simulink model "HevMmPowertrainController"  (R2021b)
settings: Solver=VariableStepAuto  StartTime=0.0  StopTime=inf  FixedStep=.01  RelTol=1e-3  EnableMultiTasking=on
model workspace (MAT data in the model file):
  Active_Scenario_Index = 1
  BattChrgMax = -105500
  BattDischrgMax = 211000
  BattTempInit = 25
  Battery.SOC_LUT = [0.01 0.02 0.03 0.04 0.05 0.06 0.07 0.08 0.09 0.1 0.11 0.12 0.13 0.14 0.15 0.16 0.17 0.18 0.19 0.2 0.21 0.22 0.23 0.24 0.25 0.26 0.27 0.28 0.29 0.3 0.31 0.32 0.33 0.34 0.35 0.36 0.37 0.38 0.39 0.4 0.41 0.42 0.43 0.44 0.45 0.46 0.47 0.48 0.49 0.5 0.51 0.52 0.53 0.54 0.55 0.56 0.57 0.58 0.59 0.6 0.61 0.62 0.63 0.64 0.65 0.66 0.67 0.68 0.69 0.7 0.71 0.72 0.73 0.74 0.75 0.76 0.77 0.78 0.79 0.8 0.81 0.82 0.83 0.84 0.85 0.86 0.87 0.88 0.89 0.9 0.91 0.92 0.93 0.94 0.95 0.96 0.97 0.98 0.99 1]
  Battery.Temperature_LUT = [-10 0 25 40]
  Battery.Capacity_LUT = [4.04528301887 4.19622641509 4.8 4.73962264151]
  Battery.Em_LUT = [2.67308083891 2.74411674384 2.80408613071 2.86247711994 2.90851059763 2.94904306488 2.9829846776 3.01467102589 3.04031502638 3.06256828113 3.08180972392 3.09994219643 ... (400 elements, 100x4)]
  Battery.R0_LUT = [0.0569026752707 0.0575506938969 0.0576730924021 0.0575627404981 0.0573787336615 0.0571931123197 0.0568199985482 0.056411926464 0.0561974340667 0.0560805640861 0.0557640899305 0.055275807865 ... (400 elements, 100x4)]
  Battery.R1_LUT = [0.0035 0.0035 0.0035 0.0035 0.0035 0.0035 0.0035 0.0035 0.0035 0.0035 0.0035 0.0035 ... (400 elements, 100x4)]
  Battery.C1_LUT = [5000 5000 5000 5000 5000 5000 5000 5000 5000 5000 5000 5000 ... (400 elements, 100x4)]
  Battery.Mass = 0.047
  Battery.ThermalMass = 44
  Battery.R_bleed = 20
  Battery.h_conv = 5
  Battery.cell_area = 0.0037
  Battery.TempInit = 25
  Battery.SOCInit = 0.75
  Battery.Model = 'panasonic ncr18650bd'
  Battery.DischargeCycle_LUT = [1 5 9 13 17 21 25 29 33 37 41 45 49 53 57 61 65 69 73 77 81 85 89 93 97 101 105 109 113 117 121 125 129 133 137 141 145 149 153 157 161 165 169 173 177 181 185 189 193 197 201 205 209 213 217 221 225 229 233 237 241 245 249 253 257 261 265 269 273 277 281 285 289 293 297 301 305 309 313 317]
  Battery.deltaEm_LUT = [0 -0.363115641304 -0.600096647258 -0.689070000839 -0.76773380251 -0.846397604181 -0.926368385458 -0.992711297521 -1.05704974111 -1.12227693902 -1.19018070587 -1.25808447272 -1.31699459748 -1.35876443799 -1.40168267642 -1.44460091485 -1.48751915327 -1.5304373917 -1.57335563013 -1.62198241593 -1.67232184498 -1.71858340023 -1.76179802551 -1.8050126508 -1.84822727608 -1.8917937136 -1.93575272784 -1.97971174208 -2.02367075632 -2.06762977056 -2.11171979109 -2.15588700406 -2.19980020032 -2.24365853098 -2.28751686164 -2.33137519231 -2.37523352297 -2.41909185363 -2.45982559031 -2.49599372373 -2.53216185715 -2.56832999058 -2.604498124 -2.64066625743 -2.67683439085 -2.71300252428 -2.7491706577 -2.78367585394 -2.81632179346 -2.8483348579 -2.88034792233 -2.91236098677 -2.94437405121 -2.97638711564 -3.00840018008 -3.04041324451 -3.07260346059 -3.10359008254 -3.13082308991 -3.15805609728 -3.18528910464 -3.21252211201 -3.23975511938 -3.26698812675 -3.29422113412 -3.32122400938 -3.3463475604 -3.37152613073 -3.39670470105 -3.42188327138 -3.4470618417 -3.47224041203 -3.49938358795 -3.52900276724 -3.55862194653 -3.58824112582 -3.6178603051 -3.64748858268 -3.67711690909 -3.70674523549]
  Battery.deltaCapacity_LUT = [0 -0.860019120059 -1.71332421702 -2.0819400264 -2.45055583577 -2.81917164515 -3.18778745452 -3.48884924257 -3.7808148236 -4.07278040463 -4.36474598566 -4.6567115667 -4.91000721732 -5.08494410056 -5.2598809838 -5.43481786703 -5.60975475027 -5.78469163351 -5.95962851674 -6.13456539998 -6.30950228322 -6.47026795816 -6.62044510558 -6.77062225299 -6.92079940041 -7.07097654783 -7.22115369524 -7.37133084266 -7.52150799007 -7.67168513749 -7.82230984162 -7.97319825819 -8.12408667477 -8.27497509134 -8.42586350792 -8.57675192449 -8.72764034107 -8.87852875764 -9.01789522921 -9.13717923376 -9.25646323831 -9.37574724285 -9.4950312474 -9.61431525195 -9.73359925649 -9.85288326104 -9.97216726558 -10.0914512701 -10.2059878191 -10.3183039593 -10.4306200996 -10.5429362398 -10.65525238 -10.7675685203 -10.8798846605 -10.9922008008 -11.104516941 -11.2125891929 -11.3075699376 -11.4025506823 -11.4975314271 -11.5925121718 -11.6874929166 -11.7824736613 -11.877454406 -11.9716325175 -12.0588579537 -12.1460833899 -12.2333088261 -12.3205342623 -12.4077596986 -12.4949851348 -12.5890165008 -12.6916254178 -12.7942343349 -12.8968432519 -12.999452169 -13.102061086 -13.2046700031 -13.3072789201]
  Battery.cond_thickness = 0.001
  Battery.thermal_conductivity = 205
  BrkPrsMax = 5000000
  CellType = 1
  ChrgLmt_bpt = [1 1 1 1 1 1 1 1 0.7 0.35 0]
  ChrgSOCHi = 80
  ChrgSOCLo = 70
  DischrgLmt_bpt = [0 0.35 0.7 1 1 1 1 1 1 1 1]
  EngCltchOffTractiveForce = 3000
  EngCltchOffVehSpd = 70
  EngCltchOnTractiveForce = 2000
  EngCltchOnVehSpd = 80
  EngCltchOnWait = 5
  EngDriveRatio = 2
  FricBrakeCmd = [0 0 12 24 36 48 60]
  FricBrakeCmdBpt = [0 0.1 0.2 0.4 0.6 0.8 1]
  MaxChrgPwr = 50000
  MaxRegenPwr = 10000
  MotGbRatio = 2.45
  MotMapEff = 0
  MotSpd = [0 1600 3200 4477.56 4800 6400 8000 9600 11200 12800 14400 16000]
  MotTrq = [450 450 450 450 419.771162405 314.828371804 251.862697443 209.885581202 179.901926745 157.414185902 139.923720802 125.931348721]
  Ndiff = 3.421
  Np_Module = 31
  Ns_Module = 24
  NumModules = 4
  OverCellVoltageLimit = 4.19999980927
  RegenBrkCutOff = [0 1]
  RegenBrkSpd_bpt = [5 9]
  Rm = 0.17778
  SOC_bpt = [0 10 20 30 40 50 60 70 80 90 100]
  T_eff_bp = [0 32.1428571429 64.2857142857 96.4285714286 128.571428571 160.714285714 192.857142857 225 257.142857143 289.285714286 321.428571429 353.571428571 385.714285714 417.857142857 450]
  TestCase = 1
  Ts = 0.01
  UnderCellVoltageLimit = 2.5
  disk_abore = 0.05
  efficiency_table = [86.7  86.7  86.7  86.7  86.7  86.7  86.7  86.7  86.7  86.7  86.7  86.7  86.7  86.7  86.7; 86.7  86.7  86.7  86.7  86.7  86.7  86.7  86.7  86.7  86.7  86.7  86.7  86.7  86.7  86.7; 86.7  86.7  91.8  91.8  91.8  91.8  91.8  91.8  91.8  91.8  89.76  89.76  89.76  89.76  89.76; 86.7  86.7  93.84  93.84  93.84  93.84  93.84  93.84  93.84  93.84  93.84  91.8  91.8  91.8  91.8; 86.7  86.7  93.84  93.84  94.86  94.86  94.86  94.86  93.84  93.84  93.84  91.8  91.8  91.8  91.8; 86.7  86.7  94.86  95.88  95.88  95.88  95.88  95.88  95.88  95.88  95.88  95.88  95.88  95.88  95.88; 86.7  86.7  94.86  95.88  95.88  96.9  96.9  96.9  96.9  96.9  96.9  96.9  96.9  96.9  96.9; 86.7  86.7  94.86  95.88  95.88  96.9  96.9  96.9  96.9  96.9  96.9  96.9  96.9  96.9  96.9; 86.7  86.7  94.86  95.88  96.9  96.9  96.9  96.9  96.9  96.9  96.9  96.9  96.9  96.9  96.9; 86.7  86.7  94.86  95.88  96.9  96.9  96.9  96.9  96.9  96.9  96.9  96.9  96.9  96.9  96.9; 86.7  86.7  94.86  95.88  95.88  95.88  95.88  95.88  95.88  95.88  95.88  95.88  95.88  95.88  95.88; 86.7  86.7  91.8  93.84  94.86  94.86  94.86  94.86  94.86  94.86  94.86  94.86  94.86  94.86  94.86]
  eng.pwr = [15052.6315789 19736.8421053 24421.0526316 29105.2631579 33789.4736842 38473.6842105 43157.8947368 47842.1052632 52526.3157895 57210.5263158 61894.7368421 66578.9473684 71263.1578947 75947.3684211 80631.5789474 85315.7894737 90000]
  eng.spd = [1448.84862461 1712.99052669 1980.33600187 2249.1155588 2517.55970613 2783.89895252 3046.3638066 3303.18477703 3552.59237246 3792.81710154 4022.08947291 4238.63999523 4440.69917715 4626.49752731 4794.26555436 4942.23376695 5068.63267374]
  eng.bsfc = [256.743221884 250.98807985 246.162934447 242.291845325 239.398872138 237.508074537 236.643512177 236.829244708 238.089331783 240.447833055 243.928808176 248.556316798 254.354418575 261.347173158 269.5586402 279.012879353 289.73395027]
  eng.trq = [99.2112225513 110.02568665 117.759751017 123.57514891 128.166058939 131.971967205 135.285068696 138.308475993 141.18967656 144.040766791 146.951280713 149.9967243 153.244568751 156.75874496 160.603298419 164.845657961 169.559869104]
  eng.idle = 1448.84862461
  eng.ff = [0.00107351698039 0.00137603113953 0.00166987721613 0.00195887997755 0.00224698941392 0.00253828073811 0.00283695438574 0.00314733601519 0.00347387650759 0.00382115196682 0.00419386371951 0.00459683831506 0.00503502752559 0.005513508346 0.00603748299394 0.00661227890981 0.00724334875674]
  eng.pwrin = [46556.889434 59676.4939829 72420.1762428 84953.8108807 97448.7032942 110081.589612 123034.636693 136495.442128 150657.034239 165717.872078 181881.845427 199358.274801 218361.911444 239112.937333 261836.965174 286765.038405 314133.631195]
  gen.max_trq = 247.580645161
  gen.max_pwr = 102.101761242
  gen.spd = [0 500 1000 1500 2000 2500 3000 3500 3938.11074919 4000 4500 5000 5500 6000 6500 7000 7500 8000 8500 9000 9500 10000 10500 11000 11500 12000 12500]
  gen.trq = [247.580645161 247.580645161 247.580645161 247.580645161 247.580645161 247.580645161 247.580645161 247.580645161 247.580645161 243.75 216.666666667 195 177.272727273 162.5 150 139.285714286 130 121.875 114.705882353 108.333333333 102.631578947 97.5 92.8571428571 88.6363636364 84.7826086957 81.25 78]
  gen.trq_cp = [243.75 216.666666667 195 177.272727273 162.5 150 139.285714286 130 121.875 114.705882353 108.333333333 102.631578947 97.5 92.8571428571 88.6363636364 84.7826086957 81.25 78]
  gen.J = 0.02
  gen.damp = 0.001
  gen.Tc = 0.02
  gen.map.spdindex = [0 1000 2000 3000 3857 4000 5000 6000 7000 8000 9000 10000 11000 12000 12584]
  gen.map.trqindex = [10 25 50 75 100 125 150 175 200 225 235.201612903]
  gen.map.eff = [84  90  90  90  90  90  90  90  90  90  90  90  90  90  90; 84  90  93  95  95  95  96  95  95  95  95  93  93  93  93; 84  90  93  95  95  95  96  95  96  95  95  95  95  93  93; 84  90  93  95  95  95  96  96  96  95  95  93  95  93  93; 84  90  93  95  95  95  96  96  96  95  95  93  93  93  93; 84  88  90  93  93  95  95  96  95  93  93  93  93  93  93; 84  88  90  90  90  93  95  95  93  93  93  93  93  93  93; 84  88  90  90  90  90  93  93  93  93  93  93  93  93  93; 84  84  88  90  90  90  90  93  93  93  93  93  93  93  93; 84  84  88  90  90  90  90  93  93  93  93  93  93  93  93; 84  84  88  90  90  90  90  93  93  93  93  93  93  93  93]
  gen.m = 20
  gen.Cp = 200
  mot.max_trq = 307
  mot.max_pwr = 124
  mot.spd = [0 500 1000 1500 2000 2500 3000 3500 3857.04487493 4000 4500 5000 5500 6000 6500 7000 7500 8000 8500 9000 9500 10000 10500 11000 11500 12000 12500]
  mot.trq = [307 307 307 307 307 307 307 307 307 296.028194151 263.136172579 236.822555321 215.29323211 197.352129434 182.171196401 169.158968086 157.881703547 148.014097075 139.307385483 131.568086289 124.643450169 118.41127766 112.772645391 107.646616055 102.9663284 98.676064717 94.7290221283]
  mot.trq_cp = [296.028194151 263.136172579 236.822555321 215.29323211 197.352129434 182.171196401 169.158968086 157.881703547 148.014097075 139.307385483 131.568086289 124.643450169 118.41127766 112.772645391 107.646616055 102.9663284 98.676064717 94.7290221283]
  mot.J = 0.02
  mot.damp = 0.0001
  mot.Tc = 0.0267
  mot.map.spdindex = [0 1000 2000 3000 3857 4000 5000 6000 7000 8000 9000 10000 11000 12000 12584]
  mot.map.trqindex = [10 25 50 75 100 125 150 175 200 225 250 275 300 307]
  mot.map.eff = [84  90  90  90  90  90  90  90  90  90  90  90  90  90  90; 84  90  93  95  95  95  96  95  95  95  95  93  93  93  93; 84  90  93  95  95  95  96  95  96  95  95  95  95  93  93; 84  90  93  95  95  95  96  96  96  95  95  95  95  93  93; 84  90  93  95  95  95  96  96  96  95  95  93  93  93  90; 84  88  90  93  93  95  95  96  95  95  95  93  93  93  90; 84  88  90  90  90  93  95  95  95  93  93  93  93  93  90; 84  88  90  90  90  90  93  93  93  93  93  93  93  93  90; 84  84  88  90  90  90  93  93  93  93  93  93  93  93  90; 84  84  88  90  90  90  90  93  93  93  93  93  93  93  90; 84  84  84  90  90  90  90  93  93  93  93  93  93  93  90; 84  84  84  88  90  90  90  93  93  93  93  93  93  93  90; 84  84  84  88  88  88  90  93  93  93  93  93  93  93  90; 84  84  84  88  88  88  90  93  93  93  93  93  93  93  90]
  mot.m = 30
  mot.Cp = 200
  mu_kinetic = 0.2
  num_pads = 2
  ts = 0.1
  w_eff_bp = [0 1600 3200 4477.56 4800 6400 8000 9600 11200 12800 14400 16000]
libraries: simulink x7, slpidlib x1, autolibutils x1
settings Model: DataDictionary=HevMmPowertrainController.sldd  ModifiedByFormat=The MathWorks, Inc.  Creator=The MathWorks, Inc.  LastModifiedBy=The MathWorks, Inc.
settings SolverCC: AlgebraicLoopSolver=TrustRegion
settings DataIOCC: ReturnWorkspaceOutputs=off
settings DebuggingCC: UnderspecifiedInitializationDetection=Classic  MergeDetectMultiDrivingBlocksExec=none  SFNoUnconditionalDefaultTransitionDiag=warning  SFMachineParentedDataDiag=warning  ArithmeticOperatorsInVariantConditions=warning
settings SFSimCC: SimUseLocalCustomCode=off
settings RTWCC: RTWUseLocalCustomCode=off
settings CodeAppCC: StateflowObjectComments=on
settings GRTTargetCC: TargetLangStandard=C89/C90 (ANSI)
settings ConfigComp: CovMetricSettings=dsw  CovSaveCumulativeToWorkspaceVar=on  CovSaveSingleToWorkspaceVar=on  CovExternalEMLEnable=off

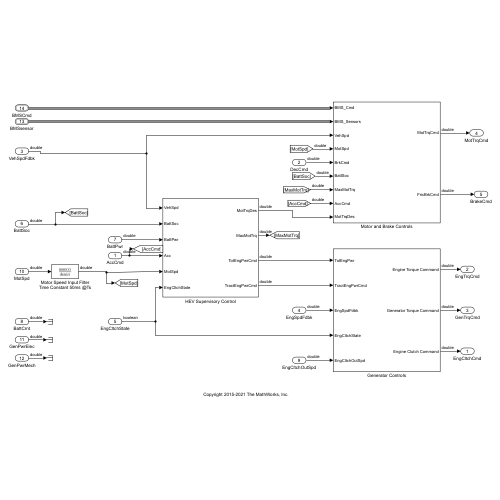
[thumbnail: Simulink's stored preview of the top-level diagram]
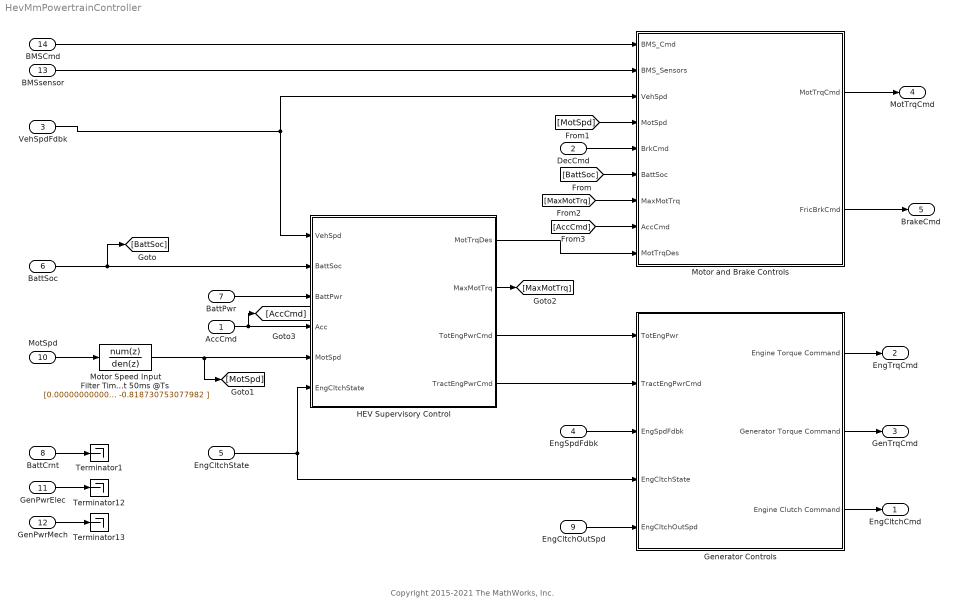
== system HevMmPowertrainController ==
  note: Copyright 2015-2021 The MathWorks, Inc.
  AccCmd : Inport
  DecCmd : Inport  Port=2  OutDataTypeStr=double
  VehSpdFdbk : Inport  Port=3
  EngSpdFdbk : Inport  Port=4
  EngCltchState : Inport  Port=5
  BattSoc : Inport  Port=6
  BattPwr : Inport  Port=7
  BattCrnt : Inport  Port=8
  EngCltchOutSpd : Inport  Port=9
  MotSpd : Inport  Port=10
  GenPwrElec : Inport  Port=11
  GenPwrMech : Inport  Port=12
  BMSsensor : Inport  Port=13  OutDataTypeStr=Bus: Sensors
  BMSCmd : Inport  Port=14  OutDataTypeStr=Bus: BMS_Cmd
  Generator Controls : Subsystem
  HEV Supervisory Control : Subsystem
  Motor Speed Input Filter Time Constant 50ms @Ts : DiscreteTransferFcn  Numerator=[0.000000000000000 0.181269246922018 ]  Denominator=[1.000000000000000 -0.818730753077982 ]  mask(DiscretizedDiscreteTransferFcn){}
      mask init:
      | %zoh
  Motor and Brake Controls : Subsystem
  Terminator1 : Terminator
  Terminator12 : Terminator
  Terminator13 : Terminator
  EngCltchCmd : Outport  VectorParamsAs1DForOutWhenUnconnected=off
  EngTrqCmd : Outport  Port=2  VectorParamsAs1DForOutWhenUnconnected=off
  GenTrqCmd : Outport  Port=3  VectorParamsAs1DForOutWhenUnconnected=off
  MotTrqCmd : Outport  Port=4  VectorParamsAs1DForOutWhenUnconnected=off
  BrakeCmd : Outport  Port=5  VectorParamsAs1DForOutWhenUnconnected=off
  wires:
  BattCrnt/1 -> Terminator1/1
  Motor and Brake Controls/1(MotTrqCmd) -> MotTrqCmd/1
  VehSpdFdbk/1 -> Motor and Brake Controls/3(VehSpd), HEV Supervisory Control/1(VehSpd)
  DecCmd/1 -> Motor and Brake Controls/5(BrkCmd)
  EngCltchState/1 -> HEV Supervisory Control/6(EngCltchState), Generator Controls/4(EngCltchState)
  HEV Supervisory Control/1(MotTrqDes) -> Motor and Brake Controls/9(MotTrqDes)
  Generator Controls/3(Engine Clutch Command) -> EngCltchCmd/1
  Motor and Brake Controls/2(FricBrkCmd) -> BrakeCmd/1
  [MotSpd] -> Motor and Brake Controls/4(MotSpd)
  EngCltchOutSpd/1 -> Generator Controls/5(EngCltchOutSpd)
  BattSoc/1 -> [BattSoc], HEV Supervisory Control/2(BattSoc)
  Motor Speed Input Filter Time Constant 50ms @Ts/1 -> [MotSpd], HEV Supervisory Control/5(MotSpd)
  [BattSoc] -> Motor and Brake Controls/6(BattSoc)
  Generator Controls/2(Generator Torque Command) -> GenTrqCmd/1
  EngSpdFdbk/1 -> Generator Controls/3(EngSpdFdbk)
  BattPwr/1 -> HEV Supervisory Control/3(BattPwr)
  AccCmd/1 -> [AccCmd], HEV Supervisory Control/4(Acc)
  HEV Supervisory Control/3(TotEngPwrCmd) -> Generator Controls/1(TotEngPwr)
  Generator Controls/1(Engine Torque Command) -> EngTrqCmd/1
  HEV Supervisory Control/4(TractEngPwrCmd) -> Generator Controls/2(TractEngPwrCmd)
  GenPwrMech/1 -> Terminator13/1
  GenPwrElec/1 -> Terminator12/1
  MotSpd/1 -> Motor Speed Input Filter Time Constant 50ms @Ts/1
  HEV Supervisory Control/2(MaxMotTrq) -> [MaxMotTrq]
  [MaxMotTrq] -> Motor and Brake Controls/7(MaxMotTrq)
  [AccCmd] -> Motor and Brake Controls/8(AccCmd)
  BMSsensor/1 -> Motor and Brake Controls/2("BMS_Sensors ")
  BMSCmd/1 -> Motor and Brake Controls/1(BMS_Cmd)

== system HevMmPowertrainController/Generator Controls ==
  TotEngPwr : Inport
  TractEngPwrCmd : Inport  Port=2
  EngSpdFdbk : Inport  Port=3
  EngCltchState : Inport  Port=4
  EngCltchOutSpd : Inport  Port=5
  Data Type Conversion : DataTypeConversion  OutDataTypeStr=boolean
  Engine Speed Input Filter : DiscreteTransferFcn  Numerator=[0.000000000000000 0.181269246922018 ]  Denominator=[1.000000000000000 -0.818730753077982 ]  mask(DiscretizedDiscreteTransferFcn){}
      mask init:
      | %zoh
  Generator Power Control : Subsystem
  Engine Torque Command : Outport  VectorParamsAs1DForOutWhenUnconnected=off
  Generator Torque Command : Outport  Port=2  VectorParamsAs1DForOutWhenUnconnected=off
  Engine Clutch Command : Outport  Port=3  VectorParamsAs1DForOutWhenUnconnected=off
  wires:
  EngSpdFdbk/1 -> Engine Speed Input Filter/1
  Generator Power Control/1(Engine Torque Command) -> Engine Torque Command/1
  Generator Power Control/2(Generator Torque Command) -> Generator Torque Command/1
  Engine Speed Input Filter/1 -> Generator Power Control/1(EngSpdFdbk)
  EngCltchOutSpd/1 -> Generator Power Control/5(EngCltchOutSpd)
  Generator Power Control/3(Engine Clutch Engage) -> Engine Clutch Command/1
  TractEngPwrCmd/1 -> Generator Power Control/3(Tractive Engine Power Command)
  EngCltchState/1 -> Data Type Conversion/1
  TotEngPwr/1 -> Generator Power Control/2(Total Engine Power Command)
  Data Type Conversion/1 -> Generator Power Control/4(EngCltchState)

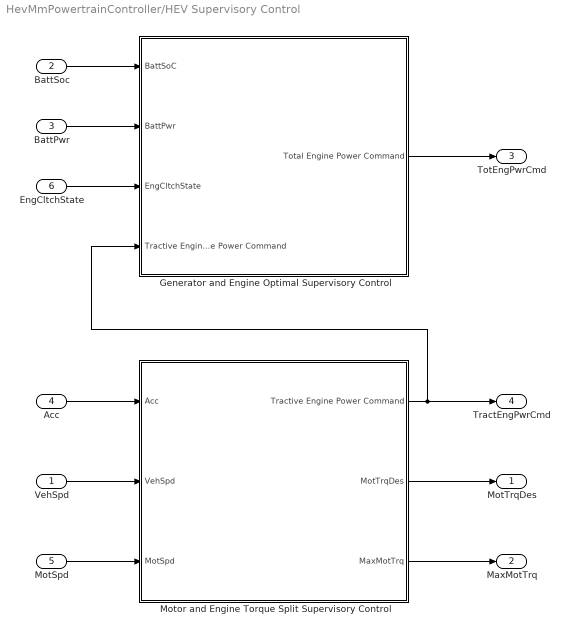
== system HevMmPowertrainController/HEV Supervisory Control ==
  VehSpd : Inport
  BattSoc : Inport  Port=2
  BattPwr : Inport  Port=3
  Acc : Inport  Port=4
  MotSpd : Inport  Port=5
  EngCltchState : Inport  Port=6
  Generator and Engine Optimal Supervisory Control : Subsystem
  Motor and Engine Torque Split Supervisory Control : Subsystem
  MotTrqDes : Outport  VectorParamsAs1DForOutWhenUnconnected=off
  MaxMotTrq : Outport  Port=2  VectorParamsAs1DForOutWhenUnconnected=off
  TotEngPwrCmd : Outport  Port=3  VectorParamsAs1DForOutWhenUnconnected=off
  TractEngPwrCmd : Outport  Port=4  VectorParamsAs1DForOutWhenUnconnected=off
  wires:
  Acc/1 -> Motor and Engine Torque Split Supervisory Control/1(Acc)
  VehSpd/1 -> Motor and Engine Torque Split Supervisory Control/2(VehSpd)
  MotSpd/1 -> Motor and Engine Torque Split Supervisory Control/3(MotSpd)
  Motor and Engine Torque Split Supervisory Control/2(MotTrqDes) -> MotTrqDes/1
  Motor and Engine Torque Split Supervisory Control/3(MaxMotTrq) -> MaxMotTrq/1
  Motor and Engine Torque Split Supervisory Control/1(Tractive Engine Power Command) -> Generator and Engine Optimal Supervisory Control/4(Tractive Engine Power Command), TractEngPwrCmd/1
  BattSoc/1 -> Generator and Engine Optimal Supervisory Control/1(BattSoC)
  BattPwr/1 -> Generator and Engine Optimal Supervisory Control/2(BattPwr)
  Generator and Engine Optimal Supervisory Control/1(Total Engine Power Command) -> TotEngPwrCmd/1
  EngCltchState/1 -> Generator and Engine Optimal Supervisory Control/3(EngCltchState)

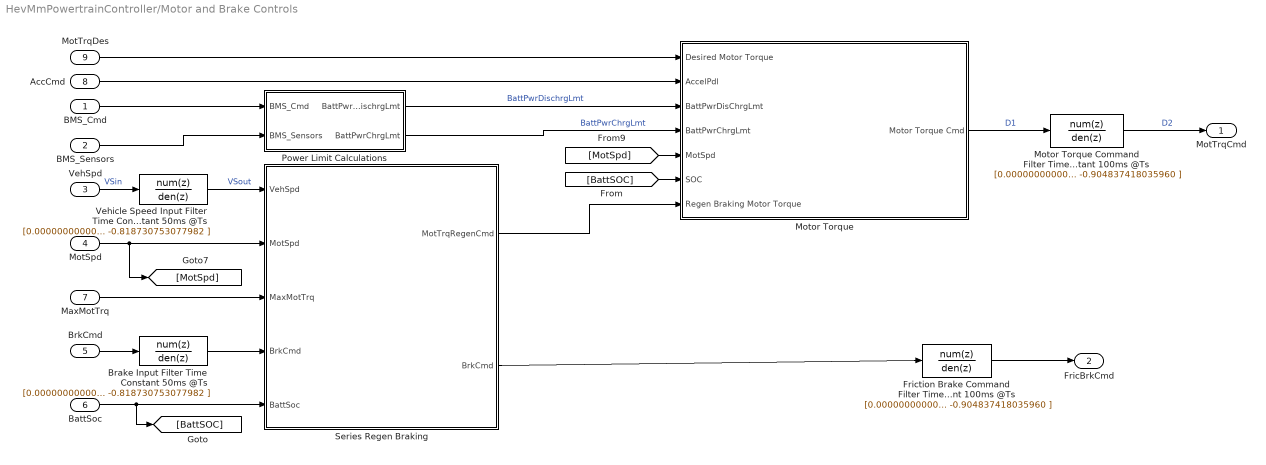
== system HevMmPowertrainController/Motor and Brake Controls ==
  BMS_Cmd : Inport
  "BMS_Sensors " : Inport  Port=2
  VehSpd : Inport  Port=3
  MotSpd : Inport  Port=4
  BrkCmd : Inport  Port=5
  BattSoc : Inport  Port=6
  MaxMotTrq : Inport  Port=7
  AccCmd : Inport  Port=8
  MotTrqDes : Inport  Port=9
  Brake Input Filter Time Constant 50ms @Ts : DiscreteTransferFcn  Numerator=[0.000000000000000 0.181269246922018 ]  Denominator=[1.000000000000000 -0.818730753077982 ]  mask(DiscretizedDiscreteTransferFcn){}
      mask init:
      | %zoh
  Friction Brake Command Filter Time constant 100ms @Ts : DiscreteTransferFcn  Numerator=[0.000000000000000 0.095162581964040 ]  Denominator=[1.000000000000000 -0.904837418035960 ]  mask(DiscretizedDiscreteTransferFcn){}
      mask init:
      | %zoh
  Motor Torque : Subsystem
  Motor Torque Command Filter Time constant 100ms @Ts : DiscreteTransferFcn  Numerator=[0.000000000000000 0.095162581964040 ]  Denominator=[1.000000000000000 -0.904837418035960 ]  mask(DiscretizedDiscreteTransferFcn){}
      mask init:
      | %zoh
  Power Limit Calculations : Subsystem
  Series Regen Braking : Subsystem  VariantControl=0
  Vehicle Speed Input Filter Time Constant 50ms @Ts : DiscreteTransferFcn  Numerator=[0.000000000000000 0.181269246922018 ]  Denominator=[1.000000000000000 -0.818730753077982 ]  mask(DiscretizedDiscreteTransferFcn){}
      mask init:
      | %zoh
  MotTrqCmd : Outport  VectorParamsAs1DForOutWhenUnconnected=off
  FricBrkCmd : Outport  Port=2  VectorParamsAs1DForOutWhenUnconnected=off
  wires:
  VehSpd/1 -> Vehicle Speed Input Filter Time Constant 50ms @Ts/1  "VSin"
  Motor Torque/1(Motor Torque Cmd) -> Motor Torque Command Filter Time constant 100ms @Ts/1  "D1"
  BrkCmd/1 -> Brake Input Filter Time Constant 50ms @Ts/1
  Series Regen Braking/1(" MotTrqRegenCmd") -> Motor Torque/7(Regen Braking Motor Torque)
  BattSoc/1 -> [BattSOC], Series Regen Braking/5(BattSoc)
  MotTrqDes/1 -> Motor Torque/1(Desired Motor Torque)
  MotSpd/1 -> [MotSpd], Series Regen Braking/2(MotSpd)
  Brake Input Filter Time Constant 50ms @Ts/1 -> Series Regen Braking/4(BrkCmd)
  Motor Torque Command Filter Time constant 100ms @Ts/1 -> MotTrqCmd/1  "D2"
  Friction Brake Command Filter Time constant 100ms @Ts/1 -> FricBrkCmd/1
  Vehicle Speed Input Filter Time Constant 50ms @Ts/1 -> Series Regen Braking/1(VehSpd)  "VSout"
  MaxMotTrq/1 -> Series Regen Braking/3(MaxMotTrq)
  Series Regen Braking/2(" BrkCmd") -> Friction Brake Command Filter Time constant 100ms @Ts/1
  AccCmd/1 -> Motor Torque/2(AccelPdl)
  [MotSpd] -> Motor Torque/5(MotSpd)
  [BattSOC] -> Motor Torque/6(SOC)
  Power Limit Calculations/1(BattPwrDischrgLmt) -> Motor Torque/3(BattPwrDisChrgLmt)  "BattPwrDischrgLmt"
  Power Limit Calculations/2(BattPwrChrgLmt) -> Motor Torque/4("BattPwrChrgLmt ")  "BattPwrChrgLmt"
  BMS_Cmd/1 -> Power Limit Calculations/1(BMS_Cmd)
  "BMS_Sensors "/1 -> Power Limit Calculations/2(BMS_Sensors)

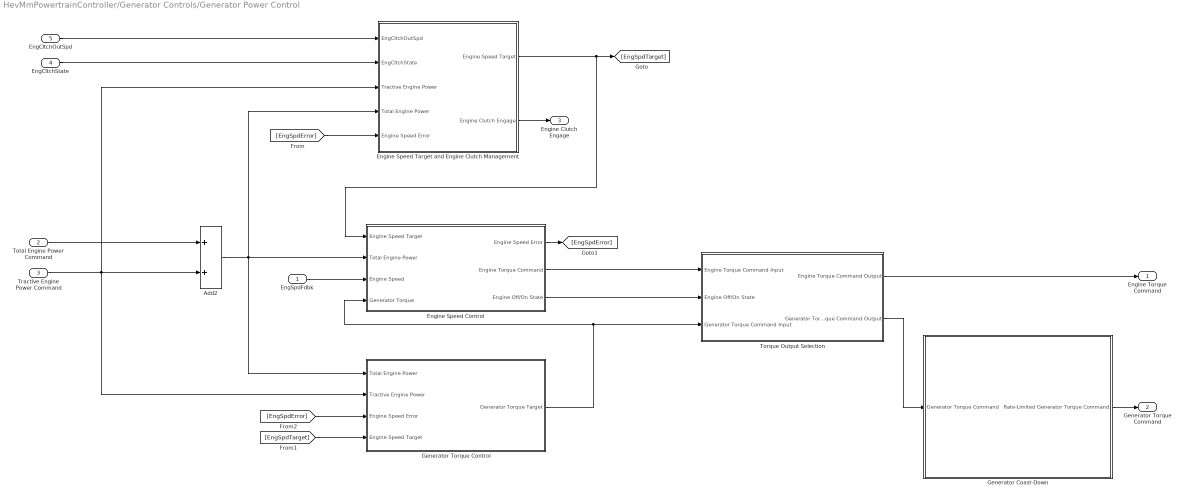
== system HevMmPowertrainController/Generator Controls/Generator Power Control ==
  EngSpdFdbk : Inport
  Total Engine Power Command : Inport  Port=2
  Tractive Engine Power Command : Inport  Port=3
  EngCltchState : Inport  Port=4
  EngCltchOutSpd : Inport  Port=5
  Add2 : Sum
  Engine Speed Control : Subsystem
  Engine Speed Target and Engine Clutch Management : Subsystem
  Generator Coast-Down : Subsystem
  Generator Torque Control : Subsystem
  Torque Output Selection : Subsystem
  Engine Torque Command : Outport  VectorParamsAs1DForOutWhenUnconnected=off
  Generator Torque Command : Outport  Port=2  VectorParamsAs1DForOutWhenUnconnected=off
  Engine Clutch Engage : Outport  Port=3  VectorParamsAs1DForOutWhenUnconnected=off
  wires:
  Add2/1 -> Engine Speed Target and Engine Clutch Management/4(Total Engine Power), Generator Torque Control/1(Total Engine Power), Engine Speed Control/2(Total Engine Power)
  Tractive Engine Power Command/1 -> Add2/2, Generator Torque Control/2(Tractive Engine Power), Engine Speed Target and Engine Clutch Management/3(Tractive Engine Power)
  Total Engine Power Command/1 -> Add2/1
  Engine Speed Target and Engine Clutch Management/1(Engine Speed Target) -> Engine Speed Control/1(Engine Speed Target), [EngSpdTarget]
  EngCltchOutSpd/1 -> Engine Speed Target and Engine Clutch Management/1(EngCltchOutSpd)
  EngCltchState/1 -> Engine Speed Target and Engine Clutch Management/2(EngCltchState)
  Engine Speed Target and Engine Clutch Management/2(Engine Clutch Engage) -> Engine Clutch Engage/1
  Engine Speed Control/3(Engine Off/On State) -> Torque Output Selection/2(Engine Off/On State)
  Engine Speed Control/1(Engine Speed Error) -> [EngSpdError]
  EngSpdFdbk/1 -> Engine Speed Control/3(Engine Speed)
  [EngSpdTarget] -> Generator Torque Control/4(Engine Speed Target)
  Generator Torque Control/1(Generator Torque Target) -> Engine Speed Control/4(Generator Torque), Torque Output Selection/3(Generator Torque Command Input)
  [EngSpdError] -> Engine Speed Target and Engine Clutch Management/5(Engine Speed Error)
  [EngSpdError] -> Generator Torque Control/3(Engine Speed Error)
  Engine Speed Control/2(Engine Torque Command) -> Torque Output Selection/1(Engine Torque Command Input)
  Torque Output Selection/2(Generator Torque Command Output) -> Generator Coast-Down/1(Generator Torque Command)
  Torque Output Selection/1(Engine Torque Command Output) -> Engine Torque Command/1
  Generator Coast-Down/1(Rate-Limited Generator Torque Command) -> Generator Torque Command/1

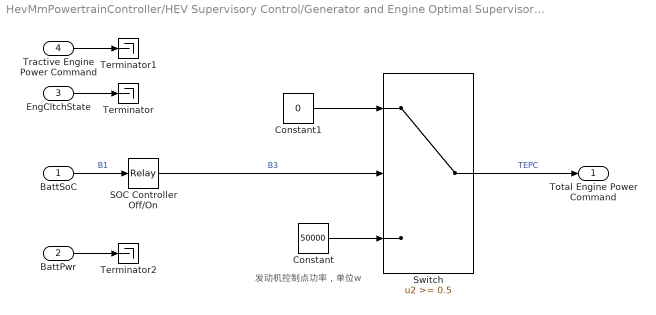
== system HevMmPowertrainController/HEV Supervisory Control/Generator and Engine Optimal Supervisory Control ==
  note: 发动机控制点功率，单位w
  BattSoC : Inport
  BattPwr : Inport  Port=2
  EngCltchState : Inport  Port=3
  Tractive Engine Power Command : Inport  Port=4
  Constant : Constant  Value=50000
  Constant1 : Constant  Value=0
  SOC Controller Off/On : Relay  OnSwitchValue=ChrgSOCHi  OffSwitchValue=ChrgSOCLo  OnOutputValue=true  OffOutputValue=false
  Switch : Switch  Threshold=0.5  ZeroCross=off
  Terminator : Terminator
  Terminator1 : Terminator
  Terminator2 : Terminator
  Total Engine Power Command : Outport  VectorParamsAs1DForOutWhenUnconnected=off
  wires:
  BattSoC/1 -> SOC Controller Off/On/1  "B1"
  EngCltchState/1 -> Terminator/1
  Tractive Engine Power Command/1 -> Terminator1/1
  BattPwr/1 -> Terminator2/1
  SOC Controller Off/On/1 -> Switch/2  "B3"
  Constant/1 -> Switch/3
  Constant1/1 -> Switch/1
  Switch/1 -> Total Engine Power Command/1  "TEPC"

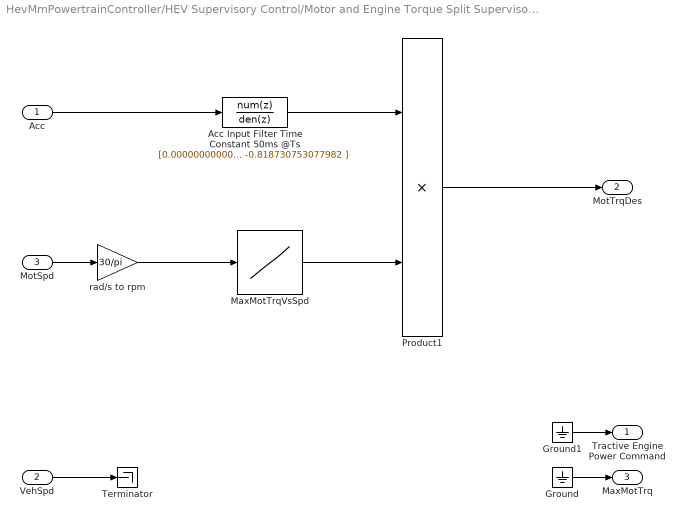
== system HevMmPowertrainController/HEV Supervisory Control/Motor and Engine Torque Split Supervisory Control ==
  Acc : Inport
  VehSpd : Inport  Port=2
  MotSpd : Inport  Port=3
  Acc Input Filter Time Constant 50ms @Ts : DiscreteTransferFcn  Numerator=[0.000000000000000 0.181269246922018 ]  Denominator=[1.000000000000000 -0.818730753077982 ]  mask(DiscretizedDiscreteTransferFcn){}
      mask init:
      | %zoh
  Ground : Ground
  Ground1 : Ground
  MaxMotTrqVsSpd : Lookup_n-D  NumberOfTableDimensions=1  BreakpointsForDimension1=MotSpd  Table=MotTrq  ExtrapMethod=Clip  UseLastTableValue=on  InternalRulePriority=Speed  OutDataTypeStr=Inherit: Inherit from 'Table data'  RndMeth=Simplest  InputSameDT=on
  Product1 : Product
  Terminator : Terminator
  rad/s to rpm : Gain  Gain=30/pi
  Tractive Engine Power Command : Outport  VectorParamsAs1DForOutWhenUnconnected=off
  MotTrqDes : Outport  Port=2  VectorParamsAs1DForOutWhenUnconnected=off
  MaxMotTrq : Outport  Port=3  VectorParamsAs1DForOutWhenUnconnected=off
  wires:
  MotSpd/1 -> rad/s to rpm/1
  Acc/1 -> Acc Input Filter Time Constant 50ms @Ts/1
  rad/s to rpm/1 -> MaxMotTrqVsSpd/1
  MaxMotTrqVsSpd/1 -> Product1/2
  Acc Input Filter Time Constant 50ms @Ts/1 -> Product1/1
  Product1/1 -> MotTrqDes/1
  Ground1/1 -> Tractive Engine Power Command/1
  VehSpd/1 -> Terminator/1
  Ground/1 -> MaxMotTrq/1

== system HevMmPowertrainController/Motor and Brake Controls/Motor Torque ==
  Desired Motor Torque : Inport
  AccelPdl : Inport  Port=2
  BattPwrDisChrgLmt : Inport  Port=3
  "BattPwrChrgLmt " : Inport  Port=4
  MotSpd : Inport  Port=5
  SOC : Inport  Port=6
  Regen Braking Motor Torque : Inport  Port=7
  Accel Decel Switch1 : Switch  Criteria=u2 > Threshold
  Compare To Constant1 : simulink/Logic and Bit Operations/Compare To Constant  relop=>  const=0  OutDataTypeStr=boolean
  Power Management : Subsystem
  Motor Torque Cmd : Outport  VectorParamsAs1DForOutWhenUnconnected=off
  wires:
  SOC/1 -> Power Management/5(SOC)
  MotSpd/1 -> Power Management/3(MotSpd)
  Desired Motor Torque/1 -> Accel Decel Switch1/1  "DMT"
  "BattPwrChrgLmt "/1 -> Power Management/2(BattPwrChrgLmt)
  BattPwrDisChrgLmt/1 -> Power Management/1(BattPwrDischrgLmt)
  Compare To Constant1/1 -> Accel Decel Switch1/2
  Power Management/1(MotTrqCmdFinal) -> Motor Torque Cmd/1
  Regen Braking Motor Torque/1 -> Accel Decel Switch1/3  "RBMT"
  Accel Decel Switch1/1 -> Power Management/4(MotTrqCmd)  "MTCin"
  AccelPdl/1 -> Compare To Constant1/1  "AccPdl"

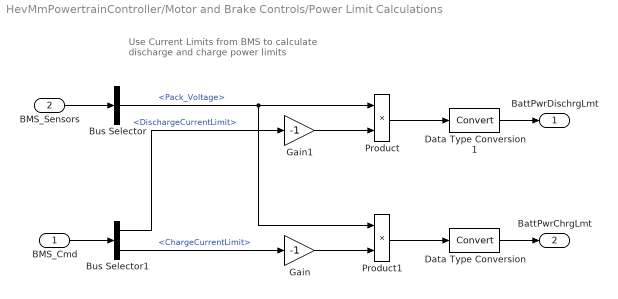
== system HevMmPowertrainController/Motor and Brake Controls/Power Limit Calculations ==
  note: Use Current Limits from BMS to calculate
      | discharge and charge power limits
  BMS_Cmd : Inport  OutDataTypeStr=Bus: BMS_Cmd
  BMS_Sensors : Inport  Port=2  OutDataTypeStr=Bus: Sensors
  Bus Selector : BusSelector  OutputSignals=Pack_Voltage
  Bus Selector1 : BusSelector  OutputSignals=CurrentLimits_Bus.DischargeCurrentLimit,CurrentLimits_Bus.ChargeCurrentLimit
  Data Type Conversion : DataTypeConversion
  Data Type Conversion1 : DataTypeConversion
  Gain : Gain  Gain=-1
  Gain1 : Gain  Gain=-1
  Product : Product
  Product1 : Product
  BattPwrDischrgLmt : Outport  VectorParamsAs1DForOutWhenUnconnected=off
  BattPwrChrgLmt : Outport  Port=2  VectorParamsAs1DForOutWhenUnconnected=off
  wires:
  Gain/1 -> Product1/2
  Gain1/1 -> Product/2
  Product/1 -> Data Type Conversion1/1
  Product1/1 -> Data Type Conversion/1
  BMS_Cmd/1 -> Bus Selector1/1
  BMS_Sensors/1 -> Bus Selector/1
  Bus Selector/1 -> Product/1, Product1/1  "<Pack_Voltage>"
  Bus Selector1/2 -> Gain/1  "<ChargeCurrentLimit>"
  Bus Selector1/1 -> Gain1/1  "<DischargeCurrentLimit>"
  Data Type Conversion/1 -> BattPwrChrgLmt/1
  Data Type Conversion1/1 -> BattPwrDischrgLmt/1

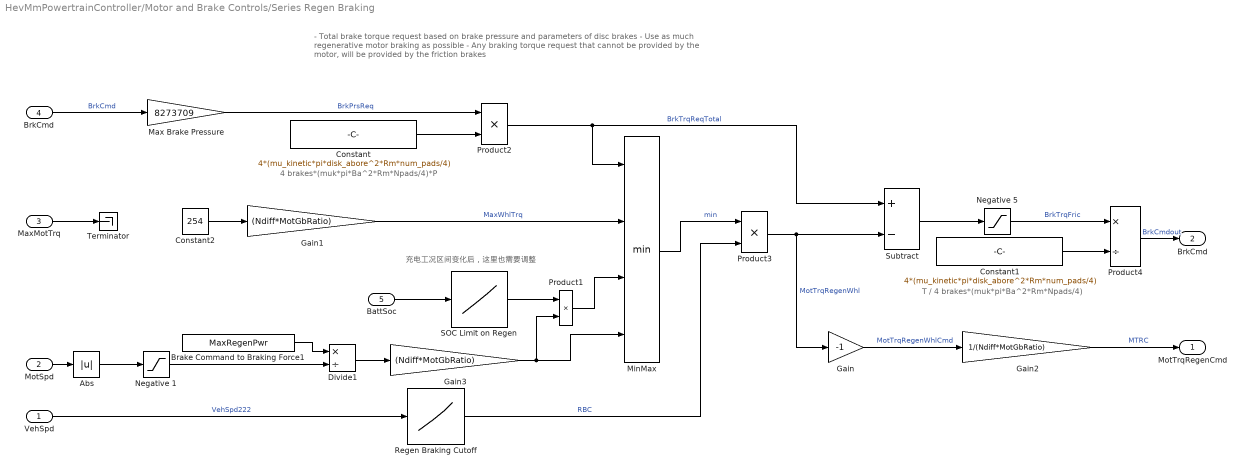
== system HevMmPowertrainController/Motor and Brake Controls/Series Regen Braking ==
  note: 充电工况区间变化后，这里也需要调整
  note: - Total brake torque request based on brake pressure and parameters of disc brakes
      | - Use as much regenerative motor braking as possible
      | -  Any braking torque request that cannot be provided by the motor, will be provided by the friction brakes
  note: T / 4 brakes*(muk*pi*Ba^2*Rm*Npads/4)
  note: 4 brakes*(muk*pi*Ba^2*Rm*Npads/4)*P
  VehSpd : Inport
  MotSpd : Inport  Port=2
  MaxMotTrq : Inport  Port=3
  BrkCmd : Inport  Port=4
  BattSoc : Inport  Port=5
  Abs : Abs  ZeroCross=off
  Brake Command to Braking Force1 : Constant  Value=MaxRegenPwr
  Constant : Constant  Value=4*(mu_kinetic*pi*disk_abore^2*Rm*num_pads/4)
  Constant1 : Constant  Value=4*(mu_kinetic*pi*disk_abore^2*Rm*num_pads/4)
  Constant2 : Constant  Value=254
  Divide1 : Product  Inputs=*/
  Gain : Gain  Gain=-1
  Gain1 : Gain  Gain=(Ndiff*MotGbRatio)
  Gain2 : Gain  Gain=1/(Ndiff*MotGbRatio)
  Gain3 : Gain  Gain=(Ndiff*MotGbRatio)
  Max Brake Pressure : Gain  Gain=8273709
  MinMax : MinMax  Inputs=4
  Negative 1 : Saturate  UpperLimit=inf  LowerLimit=1
  Negative 5 : Saturate  UpperLimit=inf  LowerLimit=0
  Product1 : Product
  Product2 : Product
  Product3 : Product
  Product4 : Product  Inputs=*/
  Regen Braking Cutoff : Lookup_n-D  NumberOfTableDimensions=1  BreakpointsForDimension1=[0.5 1]  Table=[0 1]  ExtrapMethod=Clip  InternalRulePriority=Speed  RndMeth=Simplest  InputSameDT=on
  SOC Limit on Regen : Lookup_n-D  NumberOfTableDimensions=1  BreakpointsForDimension1=[40 90]  Table=[1 0]  ExtrapMethod=Clip  InternalRulePriority=Speed  RndMeth=Simplest  InputSameDT=on
  Subtract : Sum  Inputs=+-
  Terminator : Terminator
  " MotTrqRegenCmd" : Outport  VectorParamsAs1DForOutWhenUnconnected=off
  " BrkCmd" : Outport  Port=2  VectorParamsAs1DForOutWhenUnconnected=off
  wires:
  Product3/1 -> Gain/1, Subtract/2  "MotTrqRegenWhl"
  Product4/1 -> " BrkCmd"/1  "BrkCmdout"
  Constant1/1 -> Product4/2
  Constant/1 -> Product2/2
  BrkCmd/1 -> Max Brake Pressure/1  "BrkCmd"
  MaxMotTrq/1 -> Terminator/1
  Product2/1 -> MinMax/1, Subtract/1  "BrkTrqReqTotal"
  MinMax/1 -> Product3/1  "min"
  Subtract/1 -> Negative 5/1
  Negative 5/1 -> Product4/1  "BrkTrqFric"
  Gain/1 -> Gain2/1  "MotTrqRegenWhlCmd"
  Gain1/1 -> MinMax/2  "MaxWhlTrq"
  Max Brake Pressure/1 -> Product2/1  "BrkPrsReq"
  VehSpd/1 -> Regen Braking Cutoff/1  "VehSpd222"
  Regen Braking Cutoff/1 -> Product3/2  "RBC"
  Gain2/1 -> " MotTrqRegenCmd"/1  "MTRC"
  Product1/1 -> MinMax/3
  MotSpd/1 -> Abs/1
  BattSoc/1 -> SOC Limit on Regen/1
  SOC Limit on Regen/1 -> Product1/1
  Divide1/1 -> Gain3/1
  Brake Command to Braking Force1/1 -> Divide1/1
  Abs/1 -> Negative 1/1
  Negative 1/1 -> Divide1/2
  Gain3/1 -> Product1/2, MinMax/4
  Constant2/1 -> Gain1/1

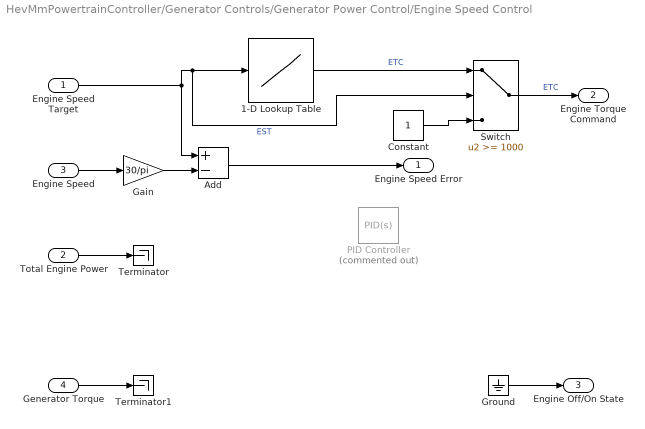
== system HevMmPowertrainController/Generator Controls/Generator Power Control/Engine Speed Control ==
  Engine Speed Target : Inport
  Total Engine Power : Inport  Port=2
  Engine Speed : Inport  Port=3
  Generator Torque : Inport  Port=4
  1-D Lookup Table : Lookup_n-D  NumberOfTableDimensions=1  BreakpointsForDimension1=eng.spd  Table=eng.trq  InternalRulePriority=Speed  RndMeth=Simplest  InputSameDT=on
  Add : Sum  Inputs=+-
  Constant : Constant  SampleTime=-1
  Gain : Gain  Gain=30/pi
  Ground : Ground
  PID Controller : slpidlib/PID Controller  Commented=on  Controller=PID  Form=Parallel  TimeDomain=Continuous-time  UseExternalTs=off  SampleTime=-1  IntegratorMethod=Forward Euler  FilterMethod=Forward Euler  ControllerParametersSource=internal  P=1  I=1  D=0  UseFilter=on  N=100  TunerSelectOption=Transfer Function Based (PID Tuner App)  InitialConditionSource=internal  InitialConditionForIntegrator=0  InitialConditionForFilter=0  DifferentiatorICPrevScaledInput=0  ExternalReset=none  TrackingMode=off  Kt=1  LimitOutput=off  SatLimitsSource=internal  UpperSaturationLimit=inf  LowerSaturationLimit=-inf  LinearizeAsGain=on  AntiWindupMode=none  Kb=1  POutMin=[]  POutMax=[]  IOutMin=[]  IOutMax=[]  DOutMin=[]  DOutMax=[]  NOutMin=[]  NOutMax=[]  SumOutMin=[]  SumOutMax=[]  SaturationOutMin=[]  SaturationOutMax=[]  PParamMin=[]  PParamMax=[]  IParamMin=[]  IParamMax=[]  DParamMin=[]  DParamMax=[]  NParamMin=[]  NParamMax=[]  KbParamMin=[]  KbParamMax=[]  KtParamMin=[]  KtParamMax=[]  KbOutMin=[]  KbOutMax=[]  KtOutMin=[]  KtOutMax=[]  IntegratorOutMin=[]  IntegratorOutMax=[]  FilterOutMin=[]  FilterOutMax=[]  SumI1OutMin=[]  SumI1OutMax=[]  SumI2OutMin=[]  SumI2OutMax=[]  SumI3OutMin=[]  SumI3OutMax=[]  SumI4OutMin=[]  SumI4OutMax=[]  SumDOutMin=[]  SumDOutMax=[]  DifferentiatorOutMin=[]  DifferentiatorOutMax=[]  FilterDiffOutCoefMin=[]  FilterDiffOutCoefMax=[]  ReciprocalOutMin=[]  ReciprocalOutMax=[]  SumDenOutMin=[]  SumDenOutMax=[]  SumNumOutMin=[]  SumNumOutMax=[]  DivideOutMin=[]  DivideOutMax=[]  UdiffTsProdOutMin=[]  UdiffTsProdOutMax=[]  NTsProdOutMin=[]  NTsProdOutMax=[]  UintegralTsProdOutMin=[]  UintegralTsProdOutMax=[]  UngainTsProdOutMin=[]  UngainTsProdOutMax=[]  IntegratorContinuousStateAttributes=''  IntegratorStateMustResolveToSignalObject=off  IntegratorRTWStateStorageClass=Auto  FilterContinuousStateAttributes=''  FilterStateMustResolveToSignalObject=off  FilterRTWStateStorageClass=Auto  ParallelPVariant=InternalParameters  IdealPVariant=Disabled  IVariant=InternalParameters  DVariant=InternalParameters  IntegratorVariant=Continuous  SatVariant=Disabled  AWVariant=Passthrough  PCopyVariant=Disabled  TRVariant=Disabled  FdbkBlocksVariant=Forward  IdealPFdbkVariant=Disabled  SatFdbkVariant=Disabled  DerivativeFilterVariant=ContFilter  NVariant=InternalParameters  NCopyVariant=Disabled  FilterICVariant=InternalICsFilter  IntegratorICVariant=InternalICs  ExternalResetVariant=Disabled  TRSumVariant=Passthrough  SumFdbkVariant=Disabled  SumVariant=Sum_PID  TsampFilterVariant=InternalTs  TsampNgainVariant=Passthrough  TsampIntegralVariant=Passthrough  ExternalSaturationOutDataTypeStr=Inherit: Same as second input
  Switch : Switch  Threshold=1000
  Terminator : Terminator
  Terminator1 : Terminator
  Engine Speed Error : Outport  VectorParamsAs1DForOutWhenUnconnected=off
  Engine Torque Command : Outport  Port=2  VectorParamsAs1DForOutWhenUnconnected=off
  Engine Off/On State : Outport  Port=3  VectorParamsAs1DForOutWhenUnconnected=off
  wires:
  Add/1 -> Engine Speed Error/1
  Engine Speed Target/1 -> Add/1, Switch/2, 1-D Lookup Table/1  "EST"
  Gain/1 -> Add/2
  Engine Speed/1 -> Gain/1
  Total Engine Power/1 -> Terminator/1
  Generator Torque/1 -> Terminator1/1
  Ground/1 -> Engine Off/On State/1
  1-D Lookup Table/1 -> Switch/1  "ETC"
  Switch/1 -> Engine Torque Command/1  "ETC"
  Constant/1 -> Switch/3

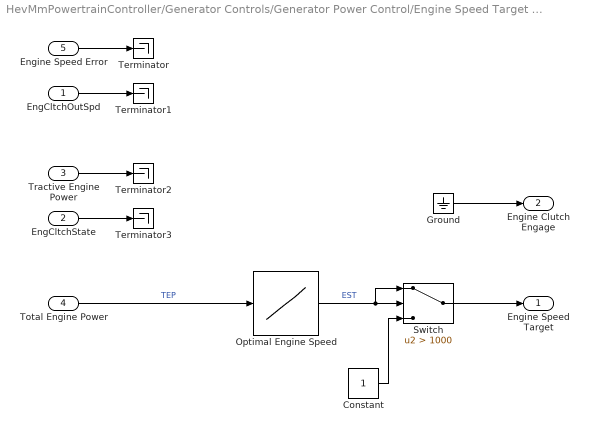
== system HevMmPowertrainController/Generator Controls/Generator Power Control/Engine Speed Target and Engine Clutch Management ==
  EngCltchOutSpd : Inport
  EngCltchState : Inport  Port=2
  Tractive Engine Power : Inport  Port=3
  Total Engine Power : Inport  Port=4
  Engine Speed Error : Inport  Port=5
  Constant : Constant  SampleTime=-1
  Ground : Ground
  Optimal Engine Speed : Lookup_n-D  NumberOfTableDimensions=1  BreakpointsForDimension1=eng.pwr  Table=eng.spd  InternalRulePriority=Speed  RndMeth=Simplest  InputSameDT=on
  Switch : Switch  Criteria=u2 > Threshold  Threshold=1000
  Terminator{,1..3} (4 alike) : Terminator
  Engine Speed Target : Outport  VectorParamsAs1DForOutWhenUnconnected=off
  Engine Clutch Engage : Outport  Port=2  VectorParamsAs1DForOutWhenUnconnected=off
  wires:
  Optimal Engine Speed/1 -> Switch/1, Switch/2  "EST"
  Total Engine Power/1 -> Optimal Engine Speed/1  "TEP"
  Engine Speed Error/1 -> Terminator/1
  EngCltchOutSpd/1 -> Terminator1/1
  Tractive Engine Power/1 -> Terminator2/1
  EngCltchState/1 -> Terminator3/1
  Ground/1 -> Engine Clutch Engage/1
  Switch/1 -> Engine Speed Target/1
  Constant/1 -> Switch/3

== system HevMmPowertrainController/Generator Controls/Generator Power Control/Generator Coast-Down ==
  Generator Torque Command : Inport
  Rate-Limited Generator Torque Command : Outport  VectorParamsAs1DForOutWhenUnconnected=off
  wires:
  Generator Torque Command/1 -> Rate-Limited Generator Torque Command/1

== system HevMmPowertrainController/Generator Controls/Generator Power Control/Generator Torque Control ==
  note: 理想功率传递无损耗
  Total Engine Power : Inport
  Tractive Engine Power : Inport  Port=2
  Engine Speed Error : Inport  Port=3
  Engine Speed Target : Inport  Port=4
  Divide : Product  Inputs=*/
  Gain : Gain  Gain=EngDriveRatio
  Terminator : Terminator
  Terminator2 : Terminator
  W to kW : Gain  Gain=1/1000*9550
  Generator Torque Target : Outport  VectorParamsAs1DForOutWhenUnconnected=off
  wires:
  Divide/1 -> Generator Torque Target/1
  Engine Speed Target/1 -> Gain/1
  Engine Speed Error/1 -> Terminator/1
  Total Engine Power/1 -> W to kW/1
  Tractive Engine Power/1 -> Terminator2/1
  W to kW/1 -> Divide/1
  Gain/1 -> Divide/2

== system HevMmPowertrainController/Generator Controls/Generator Power Control/Torque Output Selection ==
  Engine Torque Command Input : Inport
  Engine Off/On State : Inport  Port=2
  Generator Torque Command Input : Inport  Port=3
  Terminator : Terminator
  Engine Torque Command Output : Outport  VectorParamsAs1DForOutWhenUnconnected=off
  Generator Torque Command Output : Outport  Port=2  VectorParamsAs1DForOutWhenUnconnected=off
  wires:
  Generator Torque Command Input/1 -> Generator Torque Command Output/1
  Engine Torque Command Input/1 -> Engine Torque Command Output/1
  Engine Off/On State/1 -> Terminator/1

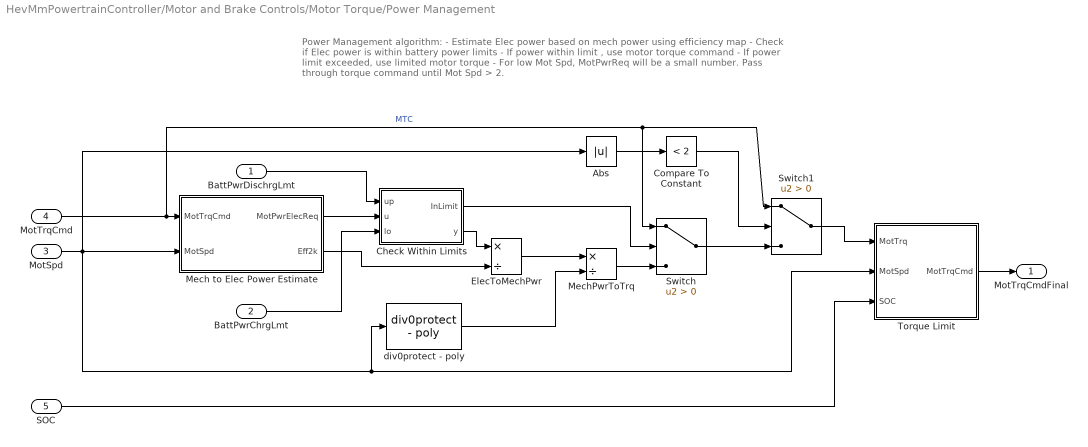
== system HevMmPowertrainController/Motor and Brake Controls/Motor Torque/Power Management ==
  note: Power Management algorithm:
      | - Estimate Elec power based on mech power using efficiency map
      | - Check if Elec power is within battery power limits
      | - If power within limit , use motor torque command
      | - If power limit exceeded, use limited motor torque
      | - For low Mot Spd, MotPwrReq will be a small number.  Pass through torque command until Mot Spd > 2.
  BattPwrDischrgLmt : Inport
  BattPwrChrgLmt : Inport  Port=2
  MotSpd : Inport  Port=3
  MotTrqCmd : Inport  Port=4
  SOC : Inport  Port=5
  Abs : Abs
  Check Within Limits : Subsystem
  Compare To Constant : simulink/Logic and Bit Operations/Compare To Constant  relop=<  const=2  OutDataTypeStr=boolean
  ElecToMechPwr : Product  Inputs=*/
  Mech to Elec Power Estimate : Subsystem
  MechPwrToTrq : Product  Inputs=*/
  Switch : Switch  Criteria=u2 > Threshold
  Switch1 : Switch  Criteria=u2 > Threshold
  Torque Limit : Subsystem
  div0protect - poly : autolibutils/div0protect - poly  thresh=2  ZeroCross1=off  aMode=aMode
      settings: SourceProductBaseCode=PW,DR,MT,UV,VE
  MotTrqCmdFinal : Outport  VectorParamsAs1DForOutWhenUnconnected=off
  wires:
  MotSpd/1 -> Abs/1, Torque Limit/2(MotSpd), div0protect - poly/1, Mech to Elec Power Estimate/2(MotSpd)
  MotTrqCmd/1 -> Switch/1, Switch1/1, Mech to Elec Power Estimate/1(MotTrqCmd)  "MTC"
  div0protect - poly/1 -> MechPwrToTrq/2
  Mech to Elec Power Estimate/2(Eff2k) -> ElecToMechPwr/2
  ElecToMechPwr/1 -> MechPwrToTrq/1
  MechPwrToTrq/1 -> Switch/3
  Torque Limit/1(MotTrqCmd) -> MotTrqCmdFinal/1
  BattPwrDischrgLmt/1 -> Check Within Limits/1(up)
  Mech to Elec Power Estimate/1(MotPwrElecReq) -> Check Within Limits/2(u)
  BattPwrChrgLmt/1 -> Check Within Limits/3(lo)
  Check Within Limits/2(y) -> ElecToMechPwr/1
  Switch/1 -> Switch1/3
  Check Within Limits/1(InLimit) -> Switch/2
  Switch1/1 -> Torque Limit/1(MotTrq)
  Abs/1 -> Compare To Constant/1
  Compare To Constant/1 -> Switch1/2
  SOC/1 -> Torque Limit/3(SOC)

== system HevMmPowertrainController/Motor and Brake Controls/Motor Torque/Power Management/Check Within Limits ==
  up : Inport
  u : Inport  Port=2
  lo : Inport  Port=3
  Compare To Zero : simulink/Logic and Bit Operations/Compare To Zero  relop=>=  OutDataTypeStr=boolean
  Compare To Zero1 : simulink/Logic and Bit Operations/Compare To Zero  relop=<=  OutDataTypeStr=boolean
  Logical Operator : Logic  AllPortsSameDT=off  OutDataTypeStr=boolean
  Saturation Dynamic1 : simulink/Discontinuities/Saturation Dynamic  OutMin=[]  OutMax=[]  OutDataTypeStr=Inherit: Same as second input  OutDataType=fixdt(1, 16)  OutScaling=2^-10  DoSatur=off
  Subtract : Sum  Inputs=+-
  Subtract1 : Sum  Inputs=-+
  InLimit : Outport  VectorParamsAs1DForOutWhenUnconnected=off
  y : Outport  Port=2  VectorParamsAs1DForOutWhenUnconnected=off
  wires:
  Saturation Dynamic1/1 -> y/1
  lo/1 -> Subtract1/2, Saturation Dynamic1/3
  up/1 -> Subtract/1, Saturation Dynamic1/1
  u/1 -> Subtract1/1, Subtract/2, Saturation Dynamic1/2
  Subtract/1 -> Compare To Zero/1
  Subtract1/1 -> Compare To Zero1/1
  Compare To Zero/1 -> Logical Operator/1
  Compare To Zero1/1 -> Logical Operator/2
  Logical Operator/1 -> InLimit/1

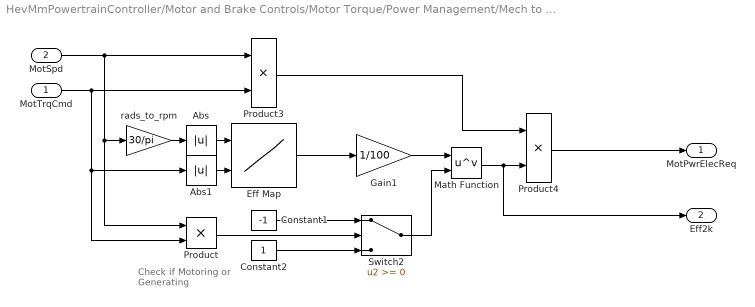
== system HevMmPowertrainController/Motor and Brake Controls/Motor Torque/Power Management/Mech to Elec Power Estimate ==
  note: Check if Motoring
      | or Generating
  MotTrqCmd : Inport
  MotSpd : Inport  Port=2
  Abs : Abs
  Abs1 : Abs
  Constant1 : Constant  Value=-1  SampleTime=-1
  Constant2 : Constant  SampleTime=-1
  Eff Map : Lookup_n-D  BreakpointsForDimension1=w_eff_bp  BreakpointsForDimension2=T_eff_bp  Table=efficiency_table  ExtrapMethod=Clip  UseLastTableValue=on  InternalRulePriority=Speed  OutDataTypeStr=Inherit: Inherit from 'Table data'  RndMeth=Simplest  InputSameDT=on
      settings: InputPortMap=u0,u1
  Gain1 : Gain  Gain=1/100
  Math Function : Math  Operator=pow  SignedPower=on  OutputSignalType=real  SaturateOnIntegerOverflow=on
  Product : Product
  Product3 : Product
  Product4 : Product
  Switch2 : Switch
  rads_to_rpm : Gain  Gain=30/pi
  MotPwrElecReq : Outport  VectorParamsAs1DForOutWhenUnconnected=off
  Eff2k : Outport  Port=2  VectorParamsAs1DForOutWhenUnconnected=off
  wires:
  Product3/1 -> Product4/1
  Switch2/1 -> Math Function/2
  Constant1/1 -> Switch2/1
  Constant2/1 -> Switch2/3
  Eff Map/1 -> Gain1/1
  Abs/1 -> Eff Map/1
  Gain1/1 -> Math Function/1
  Math Function/1 -> Eff2k/1, Product4/2
  Product4/1 -> MotPwrElecReq/1
  Abs1/1 -> Eff Map/2
  rads_to_rpm/1 -> Abs/1
  Product/1 -> Switch2/2
  MotSpd/1 -> Product3/1, Product/1, rads_to_rpm/1
  MotTrqCmd/1 -> Product3/2, Product/2, Abs1/1

== system HevMmPowertrainController/Motor and Brake Controls/Motor Torque/Power Management/Torque Limit ==
  MotTrq : Inport
  MotSpd : Inport  Port=2
  SOC : Inport  Port=3
  Compare To Constant : simulink/Logic and Bit Operations/Compare To Constant  relop=>  const=1  OutDataTypeStr=boolean
  Constant : Constant  Value=0
  Gain : Gain  Gain=-1
  MaxMotTrqVsSpd : Lookup_n-D  NumberOfTableDimensions=1  BreakpointsForDimension1=MotSpd  Table=MotTrq  ExtrapMethod=Clip  UseLastTableValue=on  InternalRulePriority=Speed  OutDataTypeStr=Inherit: Inherit from 'Table data'  RndMeth=Simplest  InputSameDT=on
  Saturation Dynamic : simulink/Discontinuities/Saturation Dynamic  OutMin=[]  OutMax=[]  OutDataTypeStr=Inherit: Same as second input  OutDataType=fixdt(1, 16)  OutScaling=2^-10  DoSatur=off
  Switch : Switch  Criteria=u2 > Threshold
  rads_to_rpm : Gain  Gain=30/pi
  MotTrqCmd : Outport  VectorParamsAs1DForOutWhenUnconnected=off
  wires:
  MotTrq/1 -> Saturation Dynamic/2  "MotTrq"
  Saturation Dynamic/1 -> MotTrqCmd/1  "MotTrqCmd"
  MotSpd/1 -> rads_to_rpm/1
  MaxMotTrqVsSpd/1 -> Gain/1, Switch/1
  rads_to_rpm/1 -> MaxMotTrqVsSpd/1
  Gain/1 -> Saturation Dynamic/3
  SOC/1 -> Compare To Constant/1
  Compare To Constant/1 -> Switch/2
  Constant/1 -> Switch/3
  Switch/1 -> Saturation Dynamic/1
